simulink model "non_linear_model"  (R2021a)
settings: Solver=VariableStepAuto  StartTime=0.0  StopTime=30  RelTol=1e-3
values from neighbouring files (symbols this model uses):
  g = 9.81    [model_structure.m]    (also in non_linear.m; pedulum_simulation.m; real_pend_sim.m)
  l = 1    [main.m]    (also in matlab.mat; non_linear.m; pedulum_simulation.m; real_pend_sim.m = 0.5)
  M = 0.5723    [model_structure.m]    (also in non_linear.m = 1; pedulum_simulation.m; real_pend_sim.m)
  m = idgrey('model_structure',par,'cd',aux,T)    [identification.m]    (also in model_structure.m = 0.12; non_linear.m = 0.5; pedulum_simulation.m = 0.12; real_pend_sim.m = 0.12)
settings Model: Creator=kpiek  LastModifiedBy=kpiek

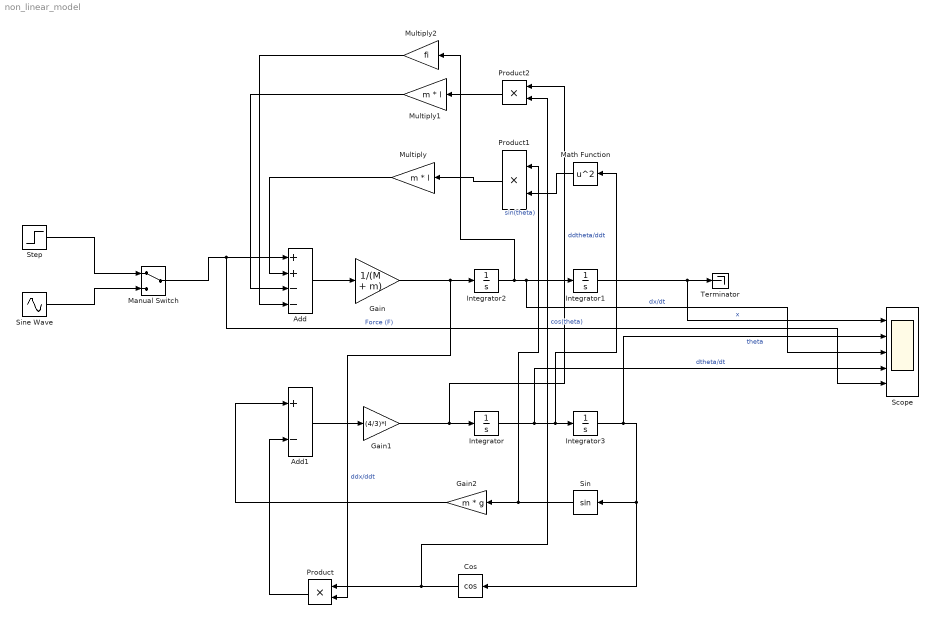
== system non_linear_model ==
  Add : Sum  Inputs=++--
  Add1 : Sum  Inputs=+-
  Cos : Trigonometry  Operator=cos
  Gain : Gain  Gain=1/(M + m)
  Gain1 : Gain  Gain=(4/3)*l
  Gain2 : Gain  Gain=m * g
  Integrator : Integrator
  Integrator1 : Integrator
  Integrator2 : Integrator
  Integrator3 : Integrator  InitialCondition=pi
  Manual Switch : ManualSwitch
  Math Function : Math  Operator=square  SaturateOnIntegerOverflow=on
  Multiply : Gain  Gain=m * l
  Multiply1 : Gain  Gain=m * l
  Multiply2 : Gain  Gain=fi
  Product : Product
  Product1 : Product
  Product2 : Product
  Scope : Scope  NumInputPorts=5
  Sin : Trigonometry
  Sine Wave : Sin  SampleTime=0
  Step : Step  SampleTime=0
  Terminator : Terminator
  wires:
  Add/1 -> Gain/1
  Gain/1 -> Product/2, Integrator2/1  "ddx/ddt"
  Add1/1 -> Gain1/1
  Gain1/1 -> Product2/1, Integrator/1  "ddtheta/ddt"
  Integrator/1 -> Scope/4, Math Function/1, Integrator3/1  "dtheta/dt"
  Integrator2/1 -> Multiply2/1, Scope/3, Integrator1/1  "dx/dt"
  Integrator1/1 -> Scope/1, Terminator/1  "x"
  Integrator3/1 -> Scope/2, Cos/1, Sin/1  "theta"
  Sin/1 -> Product1/1, Gain2/1  "sin(theta)"
  Gain2/1 -> Add1/1
  Cos/1 -> Product2/2, Product/1  "cos(theta)"
  Product/1 -> Add1/2
  Product1/1 -> Multiply/1
  Math Function/1 -> Product1/2
  Multiply/1 -> Add/2
  Product2/1 -> Multiply1/1
  Multiply1/1 -> Add/3
  Multiply2/1 -> Add/4
  Step/1 -> Manual Switch/1
  Sine Wave/1 -> Manual Switch/2
  Manual Switch/1 -> Scope/5, Add/1  "Force (F)"
